simulink model "Simulation"  (R2020b)
settings: Solver=VariableStepAuto  StartTime=0.0  StopTime=2630  MaxStep=0.1  RelTol=1e-3
values from neighbouring files (symbols this model uses):
  r2 = 23.5264    [Config.m]
undefined symbols (not defined in the file or in its folder): fs, Strejc
settings Model: Creator=Etudiants  LastModifiedBy=Etudiants

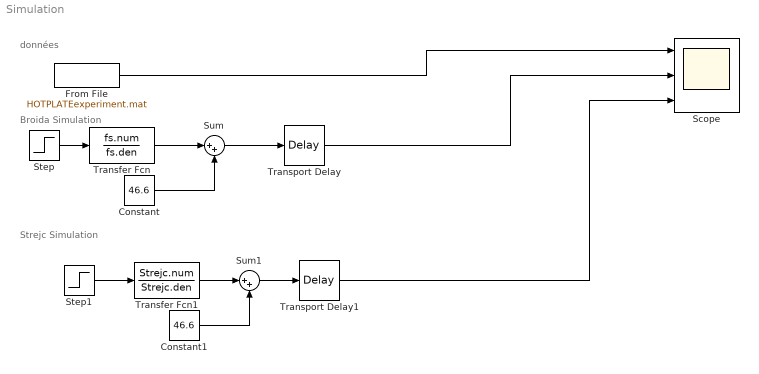
== system Simulation ==
  note: Strejc Simulation
  note: Broida Simulation
  note: données
  Constant : Constant  Value=46.6
  Constant1 : Constant  Value=46.6
  From File : FromFile  FileName=HOTPLATEexperiment.mat  SampleTime=0
  Scope : Scope  NumInputPorts=3
  Step : Step  Time=1205  After=50  SampleTime=0
  Step1 : Step  Time=1205  After=50  SampleTime=0
  Sum : Sum  Inputs=|++
  Sum1 : Sum  Inputs=|++
  Transfer Fcn : TransferFcn  Numerator=fs.num  Denominator=fs.den
  Transfer Fcn1 : TransferFcn  Numerator=Strejc.num  Denominator=Strejc.den
  Transport Delay : TransportDelay  DelayTime=9
  Transport Delay1 : TransportDelay  DelayTime=r2
  wires:
  From File/1 -> Scope/1
  Step/1 -> Transfer Fcn/1
  Transfer Fcn/1 -> Sum/1
  Constant/1 -> Sum/2
  Sum/1 -> Transport Delay/1
  Sum1/1 -> Transport Delay1/1
  Transfer Fcn1/1 -> Sum1/1
  Step1/1 -> Transfer Fcn1/1
  Constant1/1 -> Sum1/2
  Transport Delay/1 -> Scope/2
  Transport Delay1/1 -> Scope/3
